simulink model "dq2svpwm"  (R2020b)
settings: Solver=VariableStepAuto  StartTime=0.0  StopTime=0.02  RelTol=1e-3
libraries: powerlib x15, simulink x1
settings Model: Creator=Administrator  LastModifiedBy=Administrator

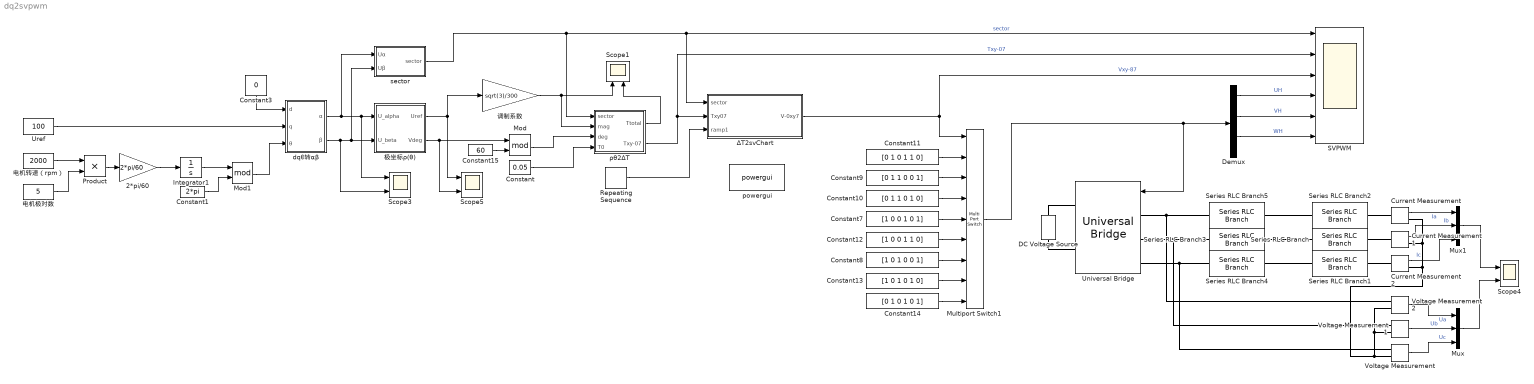
== system dq2svpwm ==
  2*pi/60 : Gain  Gain=2*pi/60
  Constant : Constant  Value=0.05
  Constant1 : Constant  Value=2*pi
  Constant10 : Constant  Value=[0 1 1 0 1 0]  VectorParams1D=off  SampleTime=-1
  Constant11 : Constant  Value=[0 1 0 1 1 0]  VectorParams1D=off  SampleTime=-1
  Constant12 : Constant  Value=[1 0 0 1 1 0]  VectorParams1D=off  SampleTime=-1
  Constant13 : Constant  Value=[1 0 1 0 1 0]  VectorParams1D=off  SampleTime=-1
  Constant14 : Constant  Value=[0 1 0 1 0 1]  VectorParams1D=off  SampleTime=-1
  Constant15 : Constant  Value=60
  Constant3 : Constant  Value=0
  Constant7 : Constant  Value=[1 0 0 1 0 1]  VectorParams1D=off  SampleTime=-1
  Constant8 : Constant  Value=[1 0 1 0 0 1]  VectorParams1D=off  SampleTime=-1
  Constant9 : Constant  Value=[0 1 1 0 0 1]  VectorParams1D=off  SampleTime=-1
  Current Measurement : powerlib/Measurements/Current Measurement  PhasorSimulation=off  OutputType=Complex  PSBequivalent=0
  Current Measurement1 : powerlib/Measurements/Current Measurement  PhasorSimulation=off  OutputType=Complex  PSBequivalent=0
  Current Measurement2 : powerlib/Measurements/Current Measurement  PhasorSimulation=off  OutputType=Complex  PSBequivalent=0
  DC Voltage Source : powerlib/Electrical Sources/DC Voltage Source  Amplitude=300  Measurements=Voltage
  Demux : Demux  Outputs=6
  Integrator1 : Integrator
  Mod : Math  Operator=mod  SaturateOnIntegerOverflow=on
  Mod1 : Math  Operator=mod  SaturateOnIntegerOverflow=on
  Multiport Switch1 : MultiPortSwitch  Inputs=8
  Mux : Mux  Inputs=3
  Mux1 : Mux  Inputs=3
  Product : Product
  Repeating Sequence : simulink/Sources/Repeating Sequence  rep_seq_t=[0 1e-4]  rep_seq_y=[0 1]
  SVPWM : Scope  NumInputPorts=6
  Scope{1,3..5} (4 alike) : Scope  NumInputPorts=2
  Series RLC Branch : powerlib/Elements/Series RLC Branch  LConnTagsString=__new0  RConnTagsString=__new0  BranchType=R  Resistance=2  Inductance=1e-3  SetiL0=off  InitialCurrent=0  Capacitance=1e-6  Setx0=off  InitialVoltage=0  Measurements=Branch current
  Series RLC Branch1 : powerlib/Elements/Series RLC Branch  LConnTagsString=__new0  RConnTagsString=__new0  BranchType=R  Resistance=2  Inductance=1e-3  SetiL0=off  InitialCurrent=0  Capacitance=1e-6  Setx0=off  InitialVoltage=0  Measurements=Branch current
  Series RLC Branch2 : powerlib/Elements/Series RLC Branch  LConnTagsString=__new0  RConnTagsString=__new0  BranchType=R  Resistance=2  Inductance=1e-3  SetiL0=off  InitialCurrent=0  Capacitance=1e-6  Setx0=off  InitialVoltage=0  Measurements=Branch current
  Series RLC Branch3 : powerlib/Elements/Series RLC Branch  LConnTagsString=__new0  RConnTagsString=__new0  BranchType=L  Resistance=2  Inductance=1e-3  SetiL0=off  InitialCurrent=0  Capacitance=1e-6  Setx0=off  InitialVoltage=0  Measurements=Branch current
  Series RLC Branch4 : powerlib/Elements/Series RLC Branch  LConnTagsString=__new0  RConnTagsString=__new0  BranchType=L  Resistance=2  Inductance=1e-3  SetiL0=off  InitialCurrent=0  Capacitance=1e-6  Setx0=off  InitialVoltage=0  Measurements=Branch current
  Series RLC Branch5 : powerlib/Elements/Series RLC Branch  LConnTagsString=__new0  RConnTagsString=__new0  BranchType=L  Resistance=2  Inductance=1e-3  SetiL0=off  InitialCurrent=0  Capacitance=1e-6  Setx0=off  InitialVoltage=0  Measurements=Branch current
  Universal Bridge : powerlib/Power Electronics/Universal Bridge  Arms=3  SnubberResistance=1e5  SnubberCapacitance=inf  Device=MOSFET / Diodes  Ron=1e-3  Lon=0  ForwardVoltages="[  50  50  ]"  ForwardVoltage=0  GTOparameters=[ 10e-6 , 20e-6 ]  IGBTparameters=[ 1e-6 , 2e-6 ]  Measurements=Device voltages  Measurements_2=None  converterType=Rectifier
  Uref : Constant  Value=100  SampleTime=1e-6
  Voltage Measurement : powerlib/Measurements/Voltage Measurement  PhasorSimulation=off  OutputType=Complex  PSBequivalent=0
  Voltage Measurement1 : powerlib/Measurements/Voltage Measurement  PhasorSimulation=off  OutputType=Complex  PSBequivalent=0
  Voltage Measurement2 : powerlib/Measurements/Voltage Measurement  PhasorSimulation=off  OutputType=Complex  PSBequivalent=0
  dqθ转αβ : Subsystem
  powergui : powerlib/powergui  Priority=1  SimulationMode=Continuous  SampleTime=50e-6  frequency=60  Iterations=50  frequencyindice=0  Pbase=100e6  ErrMax=1e-4  UnitsV=kV  UnitsW=MW  buscounter=0  FunctionMessages=off  echomessages=off  EnableUseOfTLC=off  CurrentSourceSwitches=off  DisableSnubberDevices=off  DisableRonSwitches=off  DisableVfSwitches=off  DisplayEquations=off  AutomaticDiscreteSolvers=off  SolverType=Tustin/Backward Euler (TBE)  Interpol=off  ExternalGateDelay=off  methode=off  Ts=100  x0status=blocks  SPID=on  SwTol=0  HookPort=off  NonlinearTolerance=1e-4  nMaxIteration=100  ContinueOnMaxIteration=off  RestoreLinks=warning  ResistiveCurrentMeasurement=off  Frange=[0:2:500]  Ylog=off  Xlog=on  ShowGrid=off  save=off  variable=ZData  structure=0  ZoomFFT=off  StartTime=0.0  cycles=1  DisplayStyle=1  fundamental=60  FreqAxis=off  MaxFrequency=1000  frequencyindicesteady=1  RmsSteady=1  display=off
  sector : Subsystem
  ΔT2svChart : Subsystem
  ρθ2ΔT : Subsystem
  极坐标ρ(θ) : Subsystem
  电机极对数 : Constant  Value=5  SampleTime=1e-6
  电机转速（rpm） : Constant  Value=2000  SampleTime=1e-6
  调制系数 : Gain  Gain=sqrt(3)/300
  wires:
  2*pi/60/1 -> Integrator1/1
  dqθ转αβ/1(α) -> sector/1(Uα), Scope3/1, 极坐标ρ(θ)/1("U_alpha ")
  dqθ转αβ/2(β) -> Scope3/2, 极坐标ρ(θ)/2(U_beta), sector/2(Uβ)
  Mod/1 -> ρθ2ΔT/3(deg)
  Constant8/1 -> Multiport Switch1/7
  Demux/3 -> SVPWM/5  "VH"
  Demux/5 -> SVPWM/6  "WH"
  Constant13/1 -> Multiport Switch1/8
  Demux/1 -> SVPWM/4  "UH"
  Constant9/1 -> Multiport Switch1/3
  Constant/1 -> ρθ2ΔT/4("T0 ")
  Constant10/1 -> Multiport Switch1/4
  Constant12/1 -> Multiport Switch1/6
  Constant7/1 -> Multiport Switch1/5
  ΔT2svChart/1(V-0xy7) -> SVPWM/3, Multiport Switch1/1  "Vxy-87"
  Constant11/1 -> Multiport Switch1/2
  sector/1(sector) -> ρθ2ΔT/1(sector), ΔT2svChart/1(sector), SVPWM/1  "sector"
  Constant15/1 -> Mod/2
  ρθ2ΔT/2(Txy-07) -> ΔT2svChart/2(Txy07), SVPWM/2  "Txy-07"
  Constant14/1 -> Multiport Switch1/9
  极坐标ρ(θ)/2(Vdeg) -> Scope5/2, Mod/1
  Repeating Sequence/1 -> ΔT2svChart/3(ramp1)
  Integrator1/1 -> Mod1/1
  Constant1/1 -> Mod1/2
  Mod1/1 -> dqθ转αβ/3(θ)
  Constant3/1 -> dqθ转αβ/1(d)
  Voltage Measurement2/1 -> Mux/1  "Ua"
  Voltage Measurement1/1 -> Mux/2  "Ub"
  Voltage Measurement/1 -> Mux/3  "Uc"
  Current Measurement/1 -> Mux1/1  "Ia"
  Current Measurement1/1 -> Mux1/2  "Ib"
  Current Measurement2/1 -> Mux1/3  "Ic"
  电机转速（rpm）/1 -> Product/1
  电机极对数/1 -> Product/2
  Product/1 -> 2*pi/60/1
  Uref/1 -> dqθ转αβ/2(q)
  极坐标ρ(θ)/1("Uref ") -> Scope5/1, 调制系数/1
  调制系数/1 -> ρθ2ΔT/2(mag), Scope1/1
  ρθ2ΔT/1(Ttotal) -> Scope1/2
  Mux1/1 -> Scope4/1
  Mux/1 -> Scope4/2
  Multiport Switch1/1 -> Universal Bridge/1, Demux/1
  connections:
  Current Measurement/RConn1 -- Voltage Measurement2/LConn2 -- Voltage Measurement1/LConn2 -- Voltage Measurement/LConn2 -- Current Measurement2/RConn1 -- Current Measurement1/RConn1
  DC Voltage Source/LConn1 -- Universal Bridge/RConn2
  DC Voltage Source/RConn1 -- Universal Bridge/RConn1
  Series RLC Branch5/LConn1 -- Voltage Measurement2/LConn1 -- Universal Bridge/LConn1
  Series RLC Branch3/LConn1 -- Voltage Measurement1/LConn1 -- Universal Bridge/LConn2
  Series RLC Branch4/LConn1 -- Voltage Measurement/LConn1 -- Universal Bridge/LConn3
  Series RLC Branch5/RConn1 -- Series RLC Branch2/LConn1
  Series RLC Branch2/RConn1 -- Current Measurement/LConn1
  Series RLC Branch/RConn1 -- Current Measurement1/LConn1
  Series RLC Branch1/RConn1 -- Current Measurement2/LConn1
  Series RLC Branch3/RConn1 -- Series RLC Branch/LConn1
  Series RLC Branch4/RConn1 -- Series RLC Branch1/LConn1

== system dq2svpwm/dqθ转αβ ==
  d : Inport
  q : Inport  Port=2
  θ : Inport  Port=3
  Fcn : Fcn  Expr=u(1)*sin(u(3))+u(2)*cos(u(3))
  Fcn1 : Fcn  Expr=u(1)*cos(u(3))-u(2)*sin(u(3))
  Mux : Mux  Inputs=3
  α : Outport
  β : Outport  Port=2
  wires:
  θ/1 -> Mux/3
  d/1 -> Mux/1
  Fcn1/1 -> α/1
  Fcn/1 -> β/1
  Mux/1 -> Fcn1/1, Fcn/1
  q/1 -> Mux/2

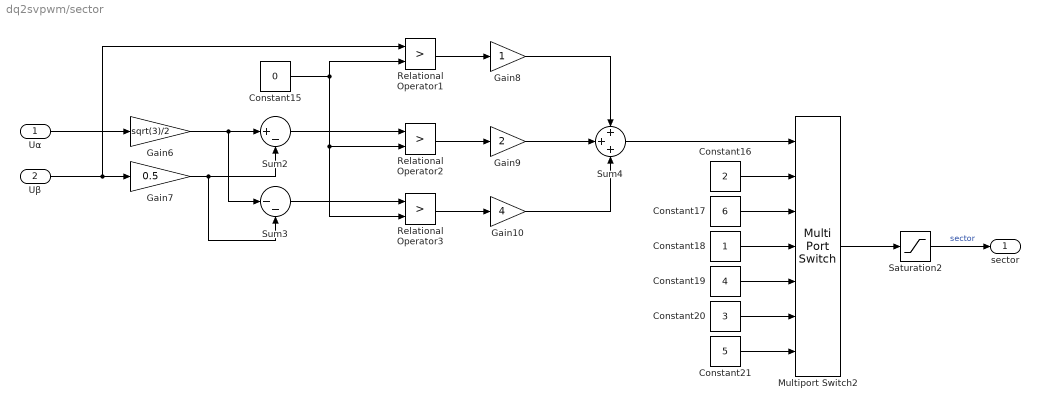
== system dq2svpwm/sector ==
  Uα : Inport
  Uβ : Inport  Port=2
  Constant15 : Constant  Value=0
  Constant16 : Constant  Value=2
  Constant17 : Constant  Value=6
  Constant18 : Constant
  Constant19 : Constant  Value=4
  Constant20 : Constant  Value=3
  Constant21 : Constant  Value=5
  Gain10 : Gain  Gain=4
  Gain6 : Gain  Gain=sqrt(3)/2
  Gain7 : Gain  Gain=0.5
  Gain8 : Gain
  Gain9 : Gain  Gain=2
  Multiport Switch2 : MultiPortSwitch  Inputs=6
  Relational Operator1 : RelationalOperator  Operator=>  OutDataTypeStr=boolean  RndMeth=Simplest
  Relational Operator2 : RelationalOperator  Operator=>  OutDataTypeStr=boolean  RndMeth=Simplest
  Relational Operator3 : RelationalOperator  Operator=>  OutDataTypeStr=boolean  RndMeth=Simplest
  Saturation2 : Saturate  UpperLimit=6  LowerLimit=1
  Sum2 : Sum  Inputs=|+-
  Sum3 : Sum  Inputs=|--
  Sum4 : Sum  Inputs=+++
  sector : Outport
  wires:
  Relational Operator1/1 -> Gain8/1
  Sum3/1 -> Relational Operator3/1
  Gain6/1 -> Sum3/1, Sum2/1
  Constant15/1 -> Relational Operator1/2, Relational Operator3/2, Relational Operator2/2
  Gain9/1 -> Sum4/2
  Uβ/1 -> Relational Operator1/1, Gain7/1
  Relational Operator3/1 -> Gain10/1
  Relational Operator2/1 -> Gain9/1
  Constant17/1 -> Multiport Switch2/3
  Constant16/1 -> Multiport Switch2/2
  Constant21/1 -> Multiport Switch2/7
  Gain10/1 -> Sum4/3
  Gain7/1 -> Sum2/2, Sum3/2
  Sum2/1 -> Relational Operator2/1
  Uα/1 -> Gain6/1
  Constant18/1 -> Multiport Switch2/4
  Constant19/1 -> Multiport Switch2/5
  Constant20/1 -> Multiport Switch2/6
  Gain8/1 -> Sum4/1
  Sum4/1 -> Multiport Switch2/1
  Multiport Switch2/1 -> Saturation2/1
  Saturation2/1 -> sector/1  "sector"

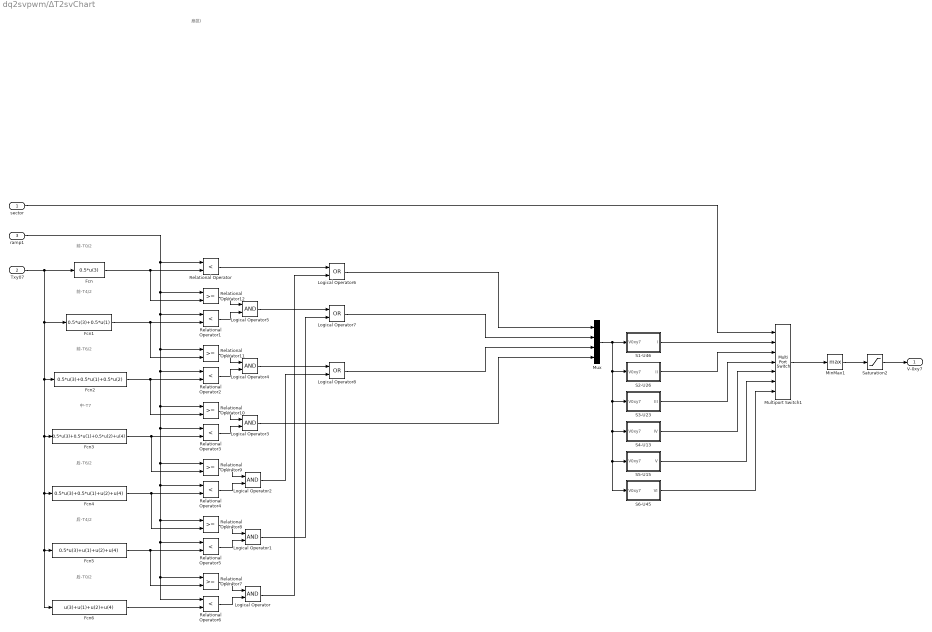
== system dq2svpwm/ΔT2svChart ==
  note: 扇区I
  note: 前-T0/2
  note: 后-T4/2
  note: 中-T7
  note: 前-T6/2
  note: 后-T0/2
  note: 前-T4/2
  note: 后-T6/2
  sector : Inport
  Txy07 : Inport  Port=2
  ramp1 : Inport  Port=3
  Fcn : Fcn  Expr=0.5*u(3)
  Fcn1 : Fcn  Expr=0.5*u(3)+0.5*u(1)
  Fcn2 : Fcn  Expr=0.5*u(3)+0.5*u(1)+0.5*u(2)
  Fcn3 : Fcn  Expr=0.5*u(3)+0.5*u(1)+0.5*u(2)+u(4)
  Fcn4 : Fcn  Expr=0.5*u(3)+0.5*u(1)+u(2)+u(4)
  Fcn5 : Fcn  Expr=0.5*u(3)+u(1)+u(2)+u(4)
  Fcn6 : Fcn  Expr=u(3)+u(1)+u(2)+u(4)
  Logical Operator{,1..5} (6 alike) : Logic  AllPortsSameDT=off  OutDataTypeStr=boolean
  Logical Operator6 : Logic  Operator=OR  AllPortsSameDT=off  OutDataTypeStr=boolean
  Logical Operator7 : Logic  Operator=OR  AllPortsSameDT=off  OutDataTypeStr=boolean
  Logical Operator8 : Logic  Operator=OR  AllPortsSameDT=off  OutDataTypeStr=boolean
  MinMax1 : MinMax  Function=max
  Multiport Switch1 : MultiPortSwitch  Inputs=6
  Mux : Mux
  Relational Operator{,1..6} (7 alike) : RelationalOperator  Operator=<  OutDataTypeStr=boolean  RndMeth=Simplest
  Relational Operator{7..12} (6 alike) : RelationalOperator  OutDataTypeStr=boolean  RndMeth=Simplest
  S1-U46 : Subsystem
  S2-U26 : Subsystem
  S3-U23 : Subsystem
  S4-U13 : Subsystem
  S5-U15 : Subsystem
  S6-U45 : Subsystem
  Saturation2 : Saturate  UpperLimit=8  LowerLimit=1
  V-0xy7 : Outport
  wires:
  Multiport Switch1/1 -> MinMax1/1
  sector/1 -> Multiport Switch1/1
  Relational Operator4/1 -> Logical Operator2/2
  Logical Operator2/1 -> Logical Operator8/2
  Logical Operator4/1 -> Logical Operator8/1
  Relational Operator7/1 -> Logical Operator/1
  Fcn5/1 -> Relational Operator7/2, Relational Operator5/2
  Relational Operator6/1 -> Logical Operator/2
  Relational Operator10/1 -> Logical Operator3/1
  Logical Operator1/1 -> Logical Operator7/2
  Relational Operator/1 -> Logical Operator6/1
  Fcn3/1 -> Relational Operator9/2, Relational Operator3/2
  Fcn4/1 -> Relational Operator8/2, Relational Operator4/2
  Relational Operator1/1 -> Logical Operator5/2
  Relational Operator11/1 -> Logical Operator4/1
  Relational Operator5/1 -> Logical Operator1/2
  Relational Operator8/1 -> Logical Operator1/1
  ramp1/1 -> Relational Operator12/1, Relational Operator11/1, Relational Operator10/1, Relational Operator9/1, Relational Operator8/1, Relational Operator7/1, Relational Operator6/1, Relational Operator5/1, Relational Operator4/1, Relational Operator3/1, Relational Operator2/1, Relational Operator1/1, Relational Operator/1
  Relational Operator9/1 -> Logical Operator2/1
  Relational Operator2/1 -> Logical Operator4/2
  Fcn1/1 -> Relational Operator11/2, Relational Operator1/2
  Fcn6/1 -> Relational Operator6/2
  Fcn2/1 -> Relational Operator10/2, Relational Operator2/2
  Logical Operator/1 -> Logical Operator6/2
  Fcn/1 -> Relational Operator12/2, Relational Operator/2
  Relational Operator3/1 -> Logical Operator3/2
  Txy07/1 -> Fcn/1, Fcn1/1, Fcn2/1, Fcn6/1, Fcn5/1, Fcn4/1, Fcn3/1
  Logical Operator6/1 -> Mux/1
  Relational Operator12/1 -> Logical Operator5/1
  Mux/1 -> S3-U23/1(V0xy7), S4-U13/1(V0xy7), S6-U45/1(V0xy7), S5-U15/1(V0xy7), S2-U26/1(V0xy7), S1-U46/1(V0xy7)
  Logical Operator3/1 -> Mux/4
  Logical Operator5/1 -> Logical Operator7/1
  S1-U46/1(I) -> Multiport Switch1/2
  S2-U26/1(II) -> Multiport Switch1/3
  S3-U23/1(III) -> Multiport Switch1/4
  S4-U13/1(IV) -> Multiport Switch1/5
  S5-U15/1(V) -> Multiport Switch1/6
  S6-U45/1(VI) -> Multiport Switch1/7
  Saturation2/1 -> V-0xy7/1
  MinMax1/1 -> Saturation2/1
  Logical Operator7/1 -> Mux/2
  Logical Operator8/1 -> Mux/3

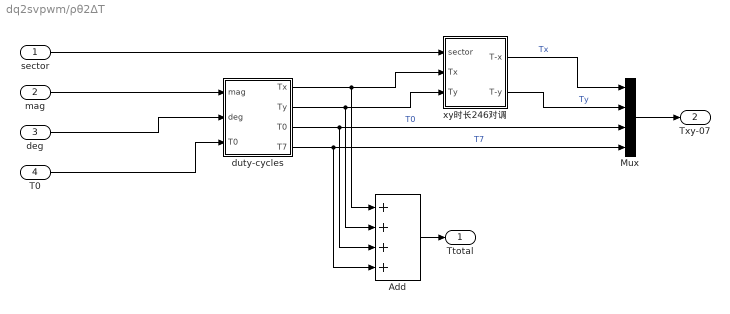
== system dq2svpwm/ρθ2ΔT ==
  sector : Inport
  mag : Inport  Port=2
  deg : Inport  Port=3
  "T0 " : Inport  Port=4
  Add : Sum  Inputs=++++
  Mux : Mux
  duty-cycles : Subsystem
  xy时长246对调 : Subsystem
  Ttotal : Outport
  Txy-07 : Outport  Port=2
  wires:
  duty-cycles/2(Ty) -> xy时长246对调/3(Ty), Add/2
  duty-cycles/4(T7) -> Add/4, Mux/4  "T7"
  deg/1 -> duty-cycles/2(deg)
  "T0 "/1 -> duty-cycles/3("T0 ")
  Mux/1 -> Txy-07/1
  duty-cycles/3(T0) -> Add/3, Mux/3  "T0"
  mag/1 -> duty-cycles/1(mag)
  duty-cycles/1(Tx) -> xy时长246对调/2(Tx), Add/1
  Add/1 -> Ttotal/1
  sector/1 -> xy时长246对调/1(sector)
  xy时长246对调/2(T-y) -> Mux/2  "Ty"
  xy时长246对调/1(T-x) -> Mux/1  "Tx"

== system dq2svpwm/极坐标ρ(θ) ==
  "U_alpha " : Inport
  U_beta : Inport  Port=2
  Gain : Gain  Gain=180/pi
  Math Function : Math  Operator=square  SignedPower=on  SaturateOnIntegerOverflow=on
  Math Function1 : Math  Operator=square  SignedPower=on  SaturateOnIntegerOverflow=on
  Sqrt : Sqrt  SaturateOnIntegerOverflow=on
  Sum : Sum  Inputs=|++
  Trigonometric Function : Trigonometry  Operator=atan2
  "Uref " : Outport
  Vdeg : Outport  Port=2
  wires:
  "U_alpha "/1 -> Math Function1/1, Trigonometric Function/2
  U_beta/1 -> Trigonometric Function/1, Math Function/1
  Math Function/1 -> Sum/1
  Math Function1/1 -> Sum/2
  Sum/1 -> Sqrt/1
  Gain/1 -> Vdeg/1
  Trigonometric Function/1 -> Gain/1
  Sqrt/1 -> "Uref "/1

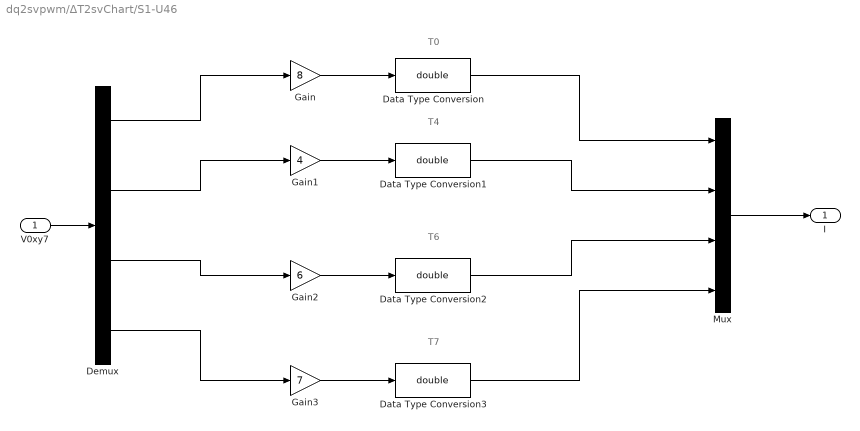
== system dq2svpwm/ΔT2svChart/S1-U46 ==
  note: T0
  note: T4
  note: T6
  note: T7
  V0xy7 : Inport
  Data Type Conversion{,1..3} (4 alike) : DataTypeConversion  OutDataTypeStr=double
  Demux : Demux
  Gain : Gain  Gain=8
  Gain1 : Gain  Gain=4
  Gain2 : Gain  Gain=6
  Gain3 : Gain  Gain=7
  Mux : Mux
  I : Outport
  wires:
  Data Type Conversion1/1 -> Mux/2
  Mux/1 -> I/1
  Gain3/1 -> Data Type Conversion3/1
  Gain1/1 -> Data Type Conversion1/1
  Data Type Conversion2/1 -> Mux/3
  Data Type Conversion/1 -> Mux/1
  Gain/1 -> Data Type Conversion/1
  Gain2/1 -> Data Type Conversion2/1
  Data Type Conversion3/1 -> Mux/4
  Demux/1 -> Gain/1
  Demux/2 -> Gain1/1
  Demux/3 -> Gain2/1
  Demux/4 -> Gain3/1
  V0xy7/1 -> Demux/1

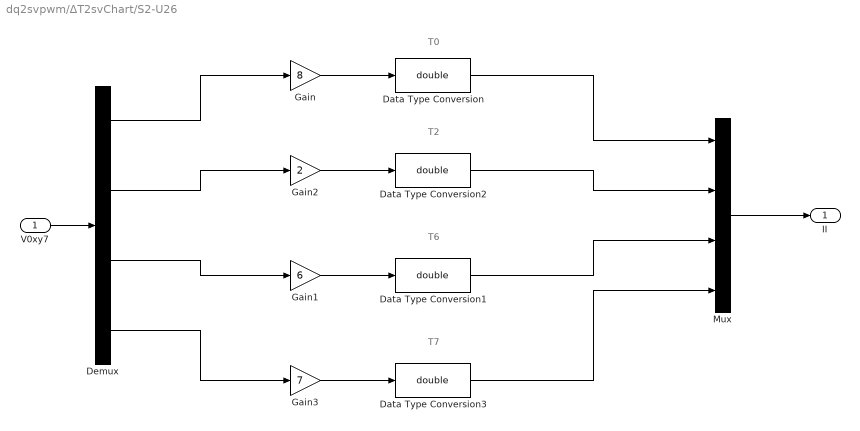
== system dq2svpwm/ΔT2svChart/S2-U26 ==
  note: T7
  note: T2
  note: T6
  note: T0
  V0xy7 : Inport
  Data Type Conversion{,1..3} (4 alike) : DataTypeConversion  OutDataTypeStr=double
  Demux : Demux
  Gain : Gain  Gain=8
  Gain1 : Gain  Gain=6
  Gain2 : Gain  Gain=2
  Gain3 : Gain  Gain=7
  Mux : Mux
  II : Outport
  wires:
  V0xy7/1 -> Demux/1
  Gain2/1 -> Data Type Conversion2/1
  Gain/1 -> Data Type Conversion/1
  Gain1/1 -> Data Type Conversion1/1
  Gain3/1 -> Data Type Conversion3/1
  Mux/1 -> II/1
  Data Type Conversion3/1 -> Mux/4
  Data Type Conversion/1 -> Mux/1
  Demux/1 -> Gain/1
  Demux/4 -> Gain3/1
  Demux/2 -> Gain2/1
  Demux/3 -> Gain1/1
  Data Type Conversion2/1 -> Mux/2
  Data Type Conversion1/1 -> Mux/3

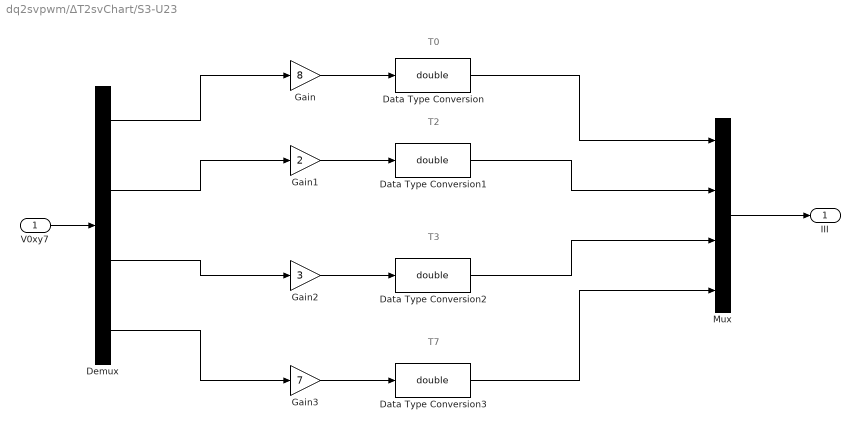
== system dq2svpwm/ΔT2svChart/S3-U23 ==
  note: T0
  note: T2
  note: T3
  note: T7
  V0xy7 : Inport
  Data Type Conversion{,1..3} (4 alike) : DataTypeConversion  OutDataTypeStr=double
  Demux : Demux
  Gain : Gain  Gain=8
  Gain1 : Gain  Gain=2
  Gain2 : Gain  Gain=3
  Gain3 : Gain  Gain=7
  Mux : Mux
  III : Outport
  wires:
  Data Type Conversion1/1 -> Mux/2
  Mux/1 -> III/1
  Gain3/1 -> Data Type Conversion3/1
  Gain1/1 -> Data Type Conversion1/1
  Data Type Conversion2/1 -> Mux/3
  Data Type Conversion/1 -> Mux/1
  Gain/1 -> Data Type Conversion/1
  Gain2/1 -> Data Type Conversion2/1
  Data Type Conversion3/1 -> Mux/4
  Demux/1 -> Gain/1
  Demux/2 -> Gain1/1
  Demux/3 -> Gain2/1
  Demux/4 -> Gain3/1
  V0xy7/1 -> Demux/1

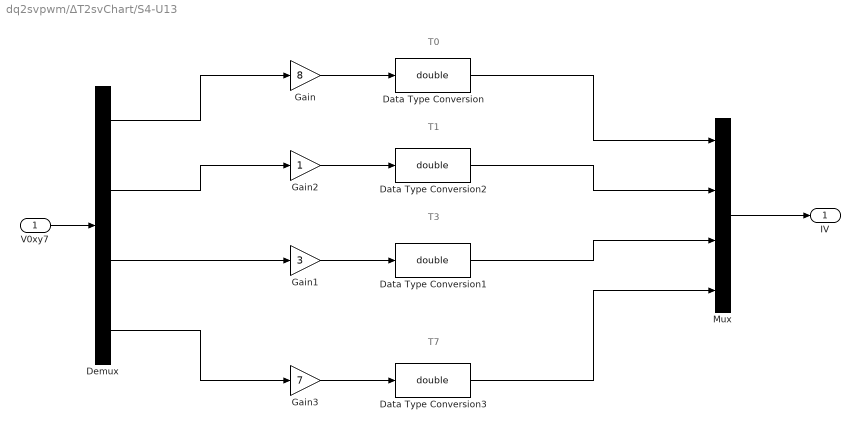
== system dq2svpwm/ΔT2svChart/S4-U13 ==
  note: T7
  note: T1
  note: T3
  note: T0
  V0xy7 : Inport
  Data Type Conversion{,1..3} (4 alike) : DataTypeConversion  OutDataTypeStr=double
  Demux : Demux
  Gain : Gain  Gain=8
  Gain1 : Gain  Gain=3
  Gain2 : Gain
  Gain3 : Gain  Gain=7
  Mux : Mux
  IV : Outport
  wires:
  V0xy7/1 -> Demux/1
  Gain2/1 -> Data Type Conversion2/1
  Gain/1 -> Data Type Conversion/1
  Gain1/1 -> Data Type Conversion1/1
  Gain3/1 -> Data Type Conversion3/1
  Mux/1 -> IV/1
  Demux/1 -> Gain/1
  Demux/4 -> Gain3/1
  Data Type Conversion/1 -> Mux/1
  Data Type Conversion3/1 -> Mux/4
  Demux/2 -> Gain2/1
  Demux/3 -> Gain1/1
  Data Type Conversion2/1 -> Mux/2
  Data Type Conversion1/1 -> Mux/3

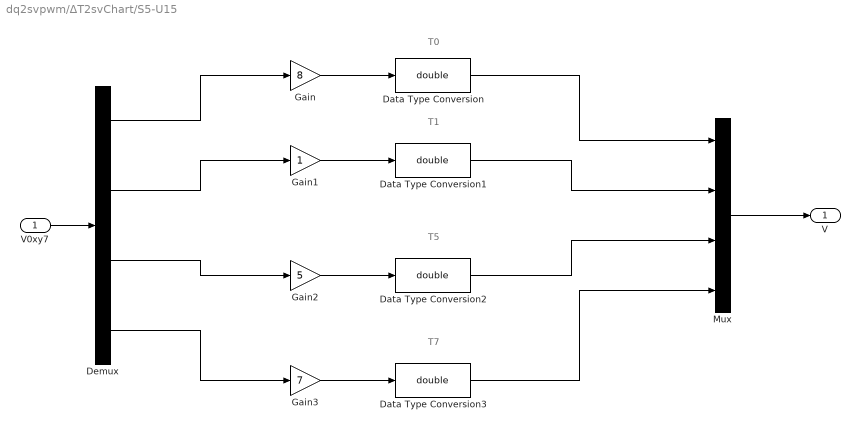
== system dq2svpwm/ΔT2svChart/S5-U15 ==
  note: T0
  note: T1
  note: T5
  note: T7
  V0xy7 : Inport
  Data Type Conversion{,1..3} (4 alike) : DataTypeConversion  OutDataTypeStr=double
  Demux : Demux
  Gain : Gain  Gain=8
  Gain1 : Gain
  Gain2 : Gain  Gain=5
  Gain3 : Gain  Gain=7
  Mux : Mux
  V : Outport
  wires:
  Data Type Conversion1/1 -> Mux/2
  Mux/1 -> V/1
  Gain3/1 -> Data Type Conversion3/1
  Gain1/1 -> Data Type Conversion1/1
  Data Type Conversion2/1 -> Mux/3
  Data Type Conversion/1 -> Mux/1
  Gain/1 -> Data Type Conversion/1
  Gain2/1 -> Data Type Conversion2/1
  Data Type Conversion3/1 -> Mux/4
  Demux/1 -> Gain/1
  Demux/2 -> Gain1/1
  Demux/3 -> Gain2/1
  Demux/4 -> Gain3/1
  V0xy7/1 -> Demux/1

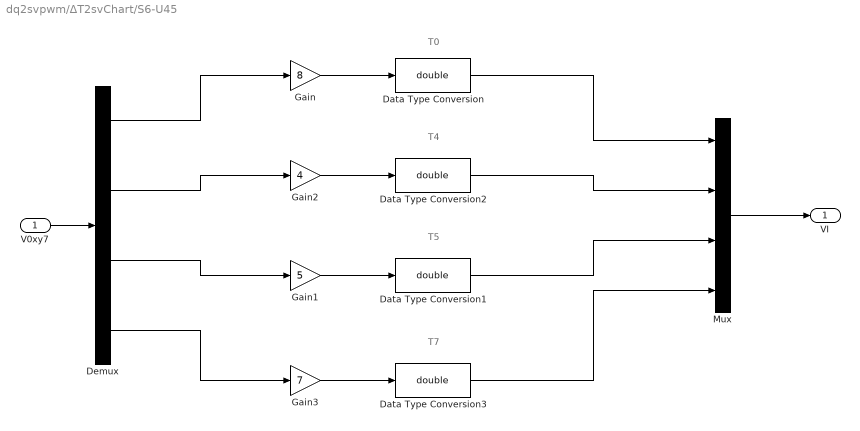
== system dq2svpwm/ΔT2svChart/S6-U45 ==
  note: T7
  note: T4
  note: T5
  note: T0
  V0xy7 : Inport
  Data Type Conversion{,1..3} (4 alike) : DataTypeConversion  OutDataTypeStr=double
  Demux : Demux
  Gain : Gain  Gain=8
  Gain1 : Gain  Gain=5
  Gain2 : Gain  Gain=4
  Gain3 : Gain  Gain=7
  Mux : Mux
  VI : Outport
  wires:
  V0xy7/1 -> Demux/1
  Gain2/1 -> Data Type Conversion2/1
  Gain/1 -> Data Type Conversion/1
  Gain1/1 -> Data Type Conversion1/1
  Gain3/1 -> Data Type Conversion3/1
  Mux/1 -> VI/1
  Data Type Conversion/1 -> Mux/1
  Demux/1 -> Gain/1
  Demux/4 -> Gain3/1
  Data Type Conversion3/1 -> Mux/4
  Demux/2 -> Gain2/1
  Demux/3 -> Gain1/1
  Data Type Conversion2/1 -> Mux/2
  Data Type Conversion1/1 -> Mux/3

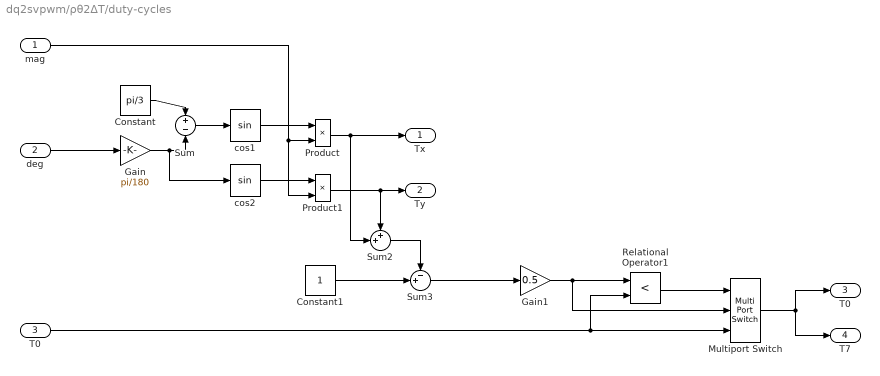
== system dq2svpwm/ρθ2ΔT/duty-cycles ==
  mag : Inport
  deg : Inport  Port=2
  "T0 " : Inport  Port=3
  Constant : Constant  Value=pi/3
  Constant1 : Constant
  Gain : Gain  Gain=pi/180
  Gain1 : Gain  Gain=0.5
  Multiport Switch : MultiPortSwitch  DataPortOrder=Zero-based contiguous  Inputs=2  zeroidx=on
  Product : Product
  Product1 : Product
  Relational Operator1 : RelationalOperator  Operator=<  OutDataTypeStr=boolean  RndMeth=Simplest
  Sum : Sum  Inputs=+|-
  Sum2 : Sum  Inputs=++|
  Sum3 : Sum  Inputs=-+|
  cos1 : Trigonometry
  cos2 : Trigonometry
  Tx : Outport
  Ty : Outport  Port=2
  T0 : Outport  Port=3
  T7 : Outport  Port=4
  wires:
  Gain/1 -> cos2/1, Sum/2
  cos1/1 -> Product/1
  Sum/1 -> cos1/1
  mag/1 -> Product1/2, Product/2
  deg/1 -> Gain/1
  Product1/1 -> Sum2/1, Ty/1
  Product/1 -> Sum2/2, Tx/1
  cos2/1 -> Product1/1
  Constant/1 -> Sum/1
  Sum2/1 -> Sum3/1
  Constant1/1 -> Sum3/2
  Sum3/1 -> Gain1/1
  Gain1/1 -> Multiport Switch/2, Relational Operator1/1
  "T0 "/1 -> Relational Operator1/2, Multiport Switch/3
  Relational Operator1/1 -> Multiport Switch/1
  Multiport Switch/1 -> T7/1, T0/1

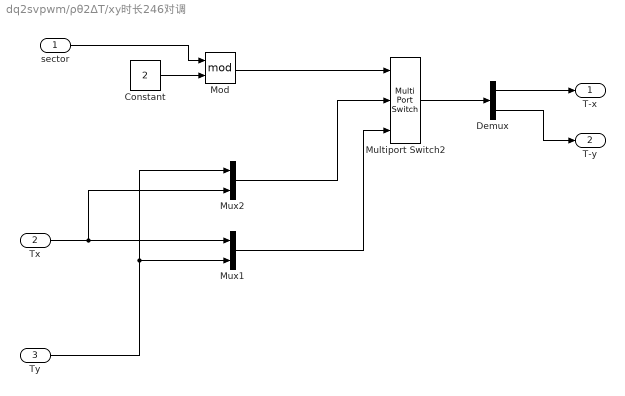
== system dq2svpwm/ρθ2ΔT/xy时长246对调 ==
  sector : Inport
  Tx : Inport  Port=2
  Ty : Inport  Port=3
  Constant : Constant  Value=2
  Demux : Demux  Outputs=2
  Mod : Math  Operator=mod  SaturateOnIntegerOverflow=on
  Multiport Switch2 : MultiPortSwitch  DataPortOrder=Zero-based contiguous  Inputs=2  zeroidx=on
  Mux1 : Mux  Inputs=2
  Mux2 : Mux  Inputs=2
  T-x : Outport
  T-y : Outport  Port=2
  wires:
  Multiport Switch2/1 -> Demux/1
  Demux/1 -> T-x/1
  Constant/1 -> Mod/2
  Mod/1 -> Multiport Switch2/1
  Tx/1 -> Mux2/2, Mux1/1
  Ty/1 -> Mux2/1, Mux1/2
  Mux1/1 -> Multiport Switch2/3
  Mux2/1 -> Multiport Switch2/2
  sector/1 -> Mod/1
  Demux/2 -> T-y/1
